simulink subsystem "Subsystem_Driver_BAv01"  (R2022b)
settings: Solver=VariableStepAuto  StartTime=0.0  StopTime=10.0  RelTol=1e-3
undefined symbols (not defined in the file): driver, param, route, weatherSim
libraries: slpidlib x2
settings Model: Creator=giaco  LastModifiedBy=giaco

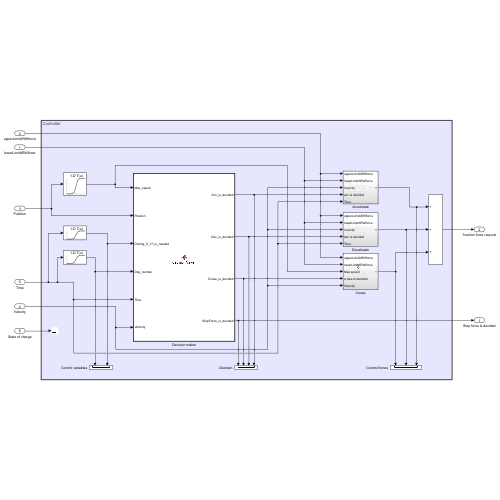
[thumbnail: Simulink's stored preview of the top-level diagram]
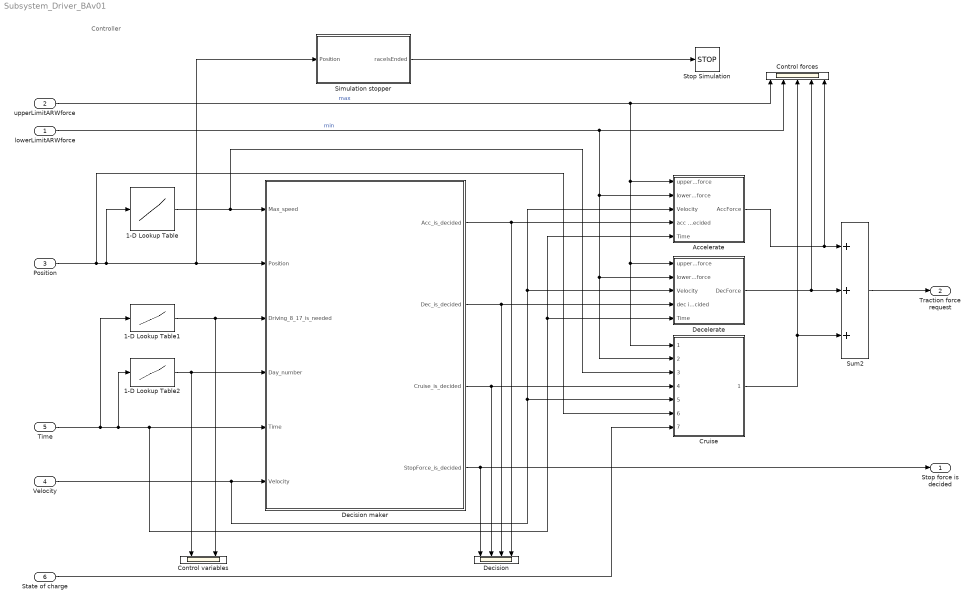
== system Subsystem_Driver_BAv01 ==
  note: Controller
  lowerLimitARWforce : Inport
  upperLimitARWforce : Inport  Port=2
  Position : Inport  Port=3
  Velocity : Inport  Port=4
  Time : Inport  Port=5
  State of charge : Inport  Port=6
  1-D Lookup Table : Lookup_n-D  NumberOfTableDimensions=1  BreakpointsForDimension1=route.dist  Table=route.maxSpeed  InternalRulePriority=Speed  RndMeth=Simplest
  1-D Lookup Table1 : Lookup_n-D  NumberOfTableDimensions=1  BreakpointsForDimension1=weatherSim.irradiance.timeSec  Table=weatherSim.irradiance.driving_8_17_Sec  InternalRulePriority=Speed
  1-D Lookup Table2 : Lookup_n-D  NumberOfTableDimensions=1  BreakpointsForDimension1=weatherSim.irradiance.timeSec  Table=weatherSim.irradiance.dayNumSec  InternalRulePriority=Speed
  Accelerate : Subsystem
  Control forces : Scope  NumInputPorts=5
  Control variables : Scope  NumInputPorts=2
  Cruise : Subsystem  ReferencedSubsystem=Subsystem_Driver_Cruise_BAv01
  Decelerate : Subsystem
  Decision : Scope  NumInputPorts=4
  Decision maker : MATLAB Function  TreatAsAtomicUnit=on
  Simulation stopper : MATLAB Function  TreatAsAtomicUnit=on
  Stop Simulation : Stop
  Sum2 : Sum  Inputs=+++
  Stop force is decided : Outport
  Traction force request : Outport  Port=2
  wires:
  Decision maker/4(StopForce_is_decided) -> Decision/1, Stop force is decided/1
  Accelerate/1(AccForce) -> Control forces/5, Sum2/1
  upperLimitARWforce/1 -> Decelerate/1(upperLimitARWforce), Cruise/1, Accelerate/1(upperLimitARWforce), Control forces/1  "max"
  Sum2/1 -> Traction force request/1
  Velocity/1 -> Decision maker/6(Velocity), Cruise/5, Accelerate/3(Velocity), Decelerate/3(Velocity)
  Decision maker/2(Dec_is_decided) -> Decision/3, Decelerate/4(dec is decided)
  Decision maker/1(Acc_is_decided) -> Decision/4, Accelerate/4(acc is decided)
  lowerLimitARWforce/1 -> Accelerate/2(lowerLimitARWforce), Decelerate/2(lowerLimitARWforce), Cruise/2, Control forces/2  "min"
  1-D Lookup Table/1 -> Decision maker/1(Max_speed), Cruise/3
  Decelerate/1(DecForce) -> Control forces/4, Sum2/2
  Time/1 -> Decision maker/5(Time), Accelerate/5(Time), Decelerate/5(Time), 1-D Lookup Table2/1, 1-D Lookup Table1/1
  Decision maker/3(Cruise_is_decided) -> Cruise/4, Decision/2
  Cruise/1 -> Control forces/3, Sum2/3
  Position/1 -> Decision maker/2(Position), Simulation stopper/1(Position), 1-D Lookup Table/1, Cruise/6
  1-D Lookup Table1/1 -> Control variables/2, Decision maker/3(Driving_8_17_is_needed)
  1-D Lookup Table2/1 -> Decision maker/4(Day_number), Control variables/1
  State of charge/1 -> Cruise/7
  Simulation stopper/1(raceIsEnded) -> Stop Simulation/1

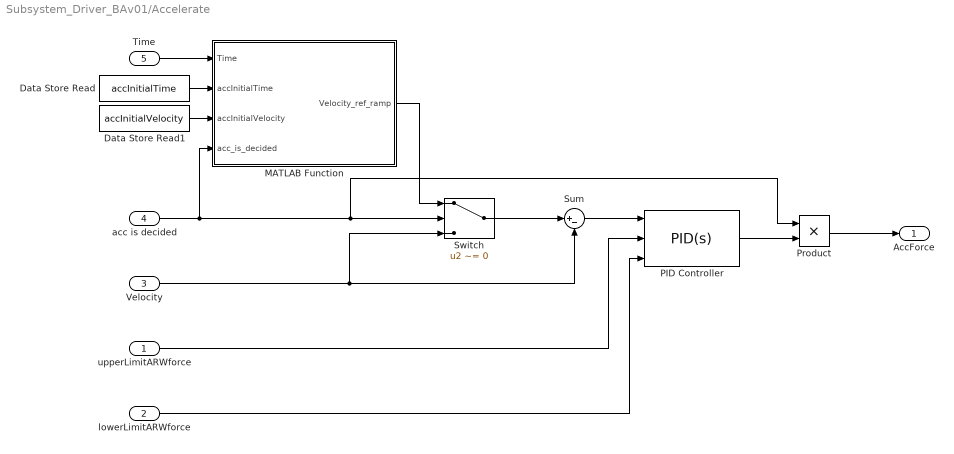
== system Subsystem_Driver_BAv01/Accelerate ==
  upperLimitARWforce : Inport
  lowerLimitARWforce : Inport  Port=2
  Velocity : Inport  Port=3
  acc is decided : Inport  Port=4
  Time : Inport  Port=5
  Data Store Read : DataStoreRead  DataStoreName=accInitialTime  IndexOptions=Index vector (dialog)  Indices=1  OutputSizes=1
  Data Store Read1 : DataStoreRead  DataStoreName=accInitialVelocity  IndexOptions=Index vector (dialog)  Indices=1  OutputSizes=1
  MATLAB Function : MATLAB Function  TreatAsAtomicUnit=on
  PID Controller : slpidlib/PID Controller  Controller=PID  Form=Ideal  TimeDomain=Continuous-time  UseExternalTs=off  SampleTime=-1  IntegratorMethod=Forward Euler  FilterMethod=Forward Euler  ControllerParametersSource=internal  P=4000  I=80/1  UseKiTs=off  D=0  N=100  UseFilter=on  TunerSelectOption=Transfer Function Based (PID Tuner App)  InitialConditionSource=internal  InitialConditionForIntegrator=0  InitialConditionForFilter=0  DifferentiatorICPrevScaledInput=0  ExternalReset=none  TrackingMode=off  Kt=1  LimitOutput=on  SatLimitsSource=external  UpperSaturationLimit=param.motor.maxTorque * param.motor.transmissionRatio / param.suspension.rWheel  LowerSaturationLimit=param.motor.minTorque * param.motor.transmissionRatio / param.suspension.rWheel  LinearizeAsGain=on  AntiWindupMode=clamping  Kb=1  LimitIntegrator=off  UpperIntegratorSaturationLimit=inf  LowerIntegratorSaturationLimit=-inf  POutMin=[]  POutMax=[]  IOutMin=[]  IOutMax=[]  DOutMin=[]  DOutMax=[]  NOutMin=[]  NOutMax=[]  SumOutMin=[]  SumOutMax=[]  SaturationOutMin=[]  SaturationOutMax=[]  PParamMin=[]  PParamMax=[]  IParamMin=[]  IParamMax=[]  DParamMin=[]  DParamMax=[]  NParamMin=[]  NParamMax=[]  KbParamMin=[]  KbParamMax=[]  KtParamMin=[]  KtParamMax=[]  KbOutMin=[]  KbOutMax=[]  KtOutMin=[]  KtOutMax=[]  IntegratorOutMin=[]  IntegratorOutMax=[]  FilterOutMin=[]  FilterOutMax=[]  SumI1OutMin=[]  SumI1OutMax=[]  SumI2OutMin=[]  SumI2OutMax=[]  SumI3OutMin=[]  SumI3OutMax=[]  SumI4OutMin=[]  SumI4OutMax=[]  SumDOutMin=[]  SumDOutMax=[]  DifferentiatorOutMin=[]  DifferentiatorOutMax=[]  FilterDiffOutCoefMin=[]  FilterDiffOutCoefMax=[]  ReciprocalOutMin=[]  ReciprocalOutMax=[]  SumDenOutMin=[]  SumDenOutMax=[]  SumNumOutMin=[]  SumNumOutMax=[]  DivideOutMin=[]  DivideOutMax=[]  UdiffTsProdOutMin=[]  UdiffTsProdOutMax=[]  NTsProdOutMin=[]  NTsProdOutMax=[]  UintegralTsProdOutMin=[]  UintegralTsProdOutMax=[]  UngainTsProdOutMin=[]  UngainTsProdOutMax=[]  ClampingZeroOutDataTypeStr=Inherit: Inherit via back propagation  ClampingZeroOutMin=[]  ClampingZeroOutMax=[]  FilterDenConstantOutDataTypeStr=Inherit: Inherit via back propagation  FilterDenConstantOutMin=[]  FilterDenConstantOutMax=[]  PCopyOutDataTypeStr=Inherit: Inherit via back propagation  PCopyOutMin=[]  PCopyOutMax=[]  NCopyOutDataTypeStr=Inherit: Inherit via back propagation  NCopyOutMin=[]  NCopyOutMax=[]  IntegratorContinuousStateAttributes=''  IntegratorStateMustResolveToSignalObject=off  IntegratorRTWStateStorageClass=Auto  FilterContinuousStateAttributes=''  FilterStateMustResolveToSignalObject=off  FilterRTWStateStorageClass=Auto  ParallelPVariant=Passthrough  IdealPVariant=InternalParameters  IVariant=InternalParameters  DVariant=InternalParameters  IntegratorVariant=Continuous  SatVariant=External  AWVariant=ContClampingIdeal  PCopyVariant=InternalParamsIdeal  TRVariant=Disabled  FdbkBlocksVariant=Forward  IdealPFdbkVariant=Disabled  SatFdbkVariant=Disabled  DerivativeFilterVariant=ContFilter  NVariant=InternalParameters  NCopyVariant=Disabled  FilterICVariant=InternalICsFilter  IntegratorICVariant=InternalICs  ExternalResetVariant=Disabled  TRSumVariant=Passthrough  SumFdbkVariant=Disabled  SumVariant=Sum_PID  TsampFilterVariant=InternalTs  TsampNgainVariant=Passthrough  TsampIntegralVariant=Passthrough  ExternalSaturationOutDataTypeStr=Inherit: Same as second input
  Product : Product
  Sum : Sum  Inputs=|+-
  Switch : Switch  Criteria=u2 ~= 0  SaturateOnIntegerOverflow=off  InputSameDT=off
  AccForce : Outport
  wires:
  acc is decided/1 -> MATLAB Function/4(acc_is_decided), Product/1, Switch/2
  Switch/1 -> Sum/1
  Velocity/1 -> Sum/2, Switch/3
  Sum/1 -> PID Controller/1
  PID Controller/1 -> Product/2
  Product/1 -> AccForce/1
  Time/1 -> MATLAB Function/1(Time)
  MATLAB Function/1(Velocity_ref_ramp) -> Switch/1
  Data Store Read/1 -> MATLAB Function/2(accInitialTime)
  Data Store Read1/1 -> MATLAB Function/3(accInitialVelocity)
  upperLimitARWforce/1 -> PID Controller/2
  lowerLimitARWforce/1 -> PID Controller/3

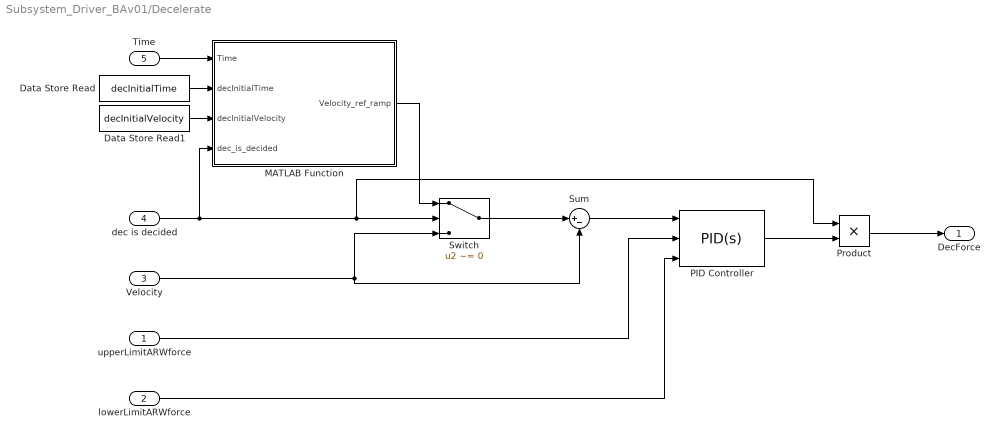
== system Subsystem_Driver_BAv01/Decelerate ==
  upperLimitARWforce : Inport
  lowerLimitARWforce : Inport  Port=2
  Velocity : Inport  Port=3
  dec is decided : Inport  Port=4
  Time : Inport  Port=5
  Data Store Read : DataStoreRead  DataStoreName=decInitialTime  IndexOptions=Index vector (dialog)  Indices=1  OutputSizes=1
  Data Store Read1 : DataStoreRead  DataStoreName=decInitialVelocity  IndexOptions=Index vector (dialog)  Indices=1  OutputSizes=1
  MATLAB Function : MATLAB Function  TreatAsAtomicUnit=on
  PID Controller : slpidlib/PID Controller  Controller=PID  Form=Ideal  TimeDomain=Continuous-time  UseExternalTs=off  SampleTime=-1  IntegratorMethod=Forward Euler  FilterMethod=Forward Euler  ControllerParametersSource=internal  P=4000  I=1/1  UseKiTs=off  D=0  N=100  UseFilter=on  TunerSelectOption=Transfer Function Based (PID Tuner App)  InitialConditionSource=internal  InitialConditionForIntegrator=0  InitialConditionForFilter=0  DifferentiatorICPrevScaledInput=0  ExternalReset=none  TrackingMode=off  Kt=1  LimitOutput=on  SatLimitsSource=external  UpperSaturationLimit=param.motor.maxTorque * param.motor.transmissionRatio / param.suspension.rWheel  LowerSaturationLimit=param.motor.minTorque * param.motor.transmissionRatio / param.suspension.rWheel  LinearizeAsGain=on  AntiWindupMode=clamping  Kb=1  LimitIntegrator=off  UpperIntegratorSaturationLimit=inf  LowerIntegratorSaturationLimit=-inf  POutMin=[]  POutMax=[]  IOutMin=[]  IOutMax=[]  DOutMin=[]  DOutMax=[]  NOutMin=[]  NOutMax=[]  SumOutMin=[]  SumOutMax=[]  SaturationOutMin=[]  SaturationOutMax=[]  PParamMin=[]  PParamMax=[]  IParamMin=[]  IParamMax=[]  DParamMin=[]  DParamMax=[]  NParamMin=[]  NParamMax=[]  KbParamMin=[]  KbParamMax=[]  KtParamMin=[]  KtParamMax=[]  KbOutMin=[]  KbOutMax=[]  KtOutMin=[]  KtOutMax=[]  IntegratorOutMin=[]  IntegratorOutMax=[]  FilterOutMin=[]  FilterOutMax=[]  SumI1OutMin=[]  SumI1OutMax=[]  SumI2OutMin=[]  SumI2OutMax=[]  SumI3OutMin=[]  SumI3OutMax=[]  SumI4OutMin=[]  SumI4OutMax=[]  SumDOutMin=[]  SumDOutMax=[]  DifferentiatorOutMin=[]  DifferentiatorOutMax=[]  FilterDiffOutCoefMin=[]  FilterDiffOutCoefMax=[]  ReciprocalOutMin=[]  ReciprocalOutMax=[]  SumDenOutMin=[]  SumDenOutMax=[]  SumNumOutMin=[]  SumNumOutMax=[]  DivideOutMin=[]  DivideOutMax=[]  UdiffTsProdOutMin=[]  UdiffTsProdOutMax=[]  NTsProdOutMin=[]  NTsProdOutMax=[]  UintegralTsProdOutMin=[]  UintegralTsProdOutMax=[]  UngainTsProdOutMin=[]  UngainTsProdOutMax=[]  ClampingZeroOutDataTypeStr=Inherit: Inherit via back propagation  ClampingZeroOutMin=[]  ClampingZeroOutMax=[]  FilterDenConstantOutDataTypeStr=Inherit: Inherit via back propagation  FilterDenConstantOutMin=[]  FilterDenConstantOutMax=[]  PCopyOutDataTypeStr=Inherit: Inherit via back propagation  PCopyOutMin=[]  PCopyOutMax=[]  NCopyOutDataTypeStr=Inherit: Inherit via back propagation  NCopyOutMin=[]  NCopyOutMax=[]  IntegratorContinuousStateAttributes=''  IntegratorStateMustResolveToSignalObject=off  IntegratorRTWStateStorageClass=Auto  FilterContinuousStateAttributes=''  FilterStateMustResolveToSignalObject=off  FilterRTWStateStorageClass=Auto  ParallelPVariant=Passthrough  IdealPVariant=InternalParameters  IVariant=InternalParameters  DVariant=InternalParameters  IntegratorVariant=Continuous  SatVariant=External  AWVariant=ContClampingIdeal  PCopyVariant=InternalParamsIdeal  TRVariant=Disabled  FdbkBlocksVariant=Forward  IdealPFdbkVariant=Disabled  SatFdbkVariant=Disabled  DerivativeFilterVariant=ContFilter  NVariant=InternalParameters  NCopyVariant=Disabled  FilterICVariant=InternalICsFilter  IntegratorICVariant=InternalICs  ExternalResetVariant=Disabled  TRSumVariant=Passthrough  SumFdbkVariant=Disabled  SumVariant=Sum_PID  TsampFilterVariant=InternalTs  TsampNgainVariant=Passthrough  TsampIntegralVariant=Passthrough  ExternalSaturationOutDataTypeStr=Inherit: Same as second input
  Product : Product
  Sum : Sum  Inputs=|+-
  Switch : Switch  Criteria=u2 ~= 0  SaturateOnIntegerOverflow=off  InputSameDT=off
  DecForce : Outport
  wires:
  dec is decided/1 -> MATLAB Function/4(dec_is_decided), Product/1, Switch/2
  Switch/1 -> Sum/1
  Velocity/1 -> Sum/2, Switch/3
  PID Controller/1 -> Product/2
  Sum/1 -> PID Controller/1
  Product/1 -> DecForce/1
  Time/1 -> MATLAB Function/1(Time)
  Data Store Read1/1 -> MATLAB Function/3(decInitialVelocity)
  MATLAB Function/1(Velocity_ref_ramp) -> Switch/1
  Data Store Read/1 -> MATLAB Function/2(decInitialTime)
  upperLimitARWforce/1 -> PID Controller/2
  lowerLimitARWforce/1 -> PID Controller/3

== matlab function Subsystem_Driver_BAv01/Accelerate/MATLAB Function ==
  data: Time input; Velocity_ref_ramp output; accInitialTime input; accInitialVelocity input; driver parameter; acc_is_decided input
function Velocity_ref_ramp = fcn(Time, accInitialTime, accInitialVelocity, driver, acc_is_decided)

Velocity_ref_ramp = 0;

if acc_is_decided
    Velocity_ref_ramp = driver.accRef .* (Time - accInitialTime) + accInitialVelocity;
end

== matlab function Subsystem_Driver_BAv01/Decelerate/MATLAB Function ==
  data: Time input; Velocity_ref_ramp output; decInitialTime input; decInitialVelocity input; driver parameter; dec_is_decided input
function Velocity_ref_ramp = fcn(Time, decInitialTime, decInitialVelocity, driver, dec_is_decided)

Velocity_ref_ramp = 0;

if dec_is_decided
    Velocity_ref_ramp = driver.decRef .* (Time - decInitialTime) + decInitialVelocity;
end

== matlab function Subsystem_Driver_BAv01/Decision maker ==
  settings: updateMethod=DISCRETE
  data: Max_speed input; Position input; Driving_8_17_is_needed input; Day_number input; Time input; Velocity input; spaceStopIsOver data_store_memory; timeStopIsNeeded data_store_memory; spaceStopIsNeeded data_store_memory; driver parameter; spaceStopNumber data_store_memory; spaceStopIsStarted data_store_memory; Acc_is_decided output; Dec_is_decided output; Cruise_is_decided output; StopForce_is_decided output; spaceStopInitialTime data_store_memory; accInitialTime data_store_memory; accInitialVelocity data_store_memory; decInitialTime data_store_memory; decInitialVelocity data_store_memory; racingDayIsStarted data_store_memory; dayNumber data_store_memory; weatherSim parameter
function [Acc_is_decided, Dec_is_decided, Cruise_is_decided, StopForce_is_decided] = decisionMaker(Max_speed, Position, Driving_8_17_is_needed, Day_number, Time, Velocity, driver, weatherSim)

global racingDayIsStarted
global timeStopIsNeeded
global dayNumber

global spaceStopIsNeeded
global spaceStopIsStarted
global spaceStopIsOver
global spaceStopInitialTime
global spaceStopNumber

global accInitialTime
global accInitialVelocity
global decInitialTime
global decInitialVelocity

Acc_is_decided = false;
Dec_is_decided = false;
Cruise_is_decided = false;
StopForce_is_decided = false;

controlVelocity = min(driver.velRef, Max_speed);

%% Check for stops
% Time stops
stopTime = Time - Velocity ./ driver.decRef;

if ~timeStopIsNeeded && stopTime >= (weatherSim.irradiance.stopTimeSec(Day_number) - 60) %to be sure to stop on time
    timeStopIsNeeded = true;
    decInitialTime = Time; %initialization of time and velocity for ramp controller
    decInitialVelocity = Velocity;
end % if

% Space stops
stopDistance = Position - Velocity.^2 / (2 * driver.decRef);

if ~spaceStopIsNeeded && stopDistance >= driver.stopLocDist(spaceStopNumber)
    spaceStopIsNeeded = true;
    decInitialTime = Time; %initialization of time and velocity for ramp controller
    decInitialVelocity = Velocity;
    
    if spaceStopNumber < length(driver.stopLocDist) %omit last stop: stop simulation
        spaceStopNumber = spaceStopNumber + 1;
    end % if
end % if

%% Check for new racing day
if Driving_8_17_is_needed && Day_number == dayNumber
    racingDayIsStarted = true;
    timeStopIsNeeded = false;
    dayNumber = dayNumber + 1;
end % if

%% Select control options
%% Deceleration
if timeStopIsNeeded
    if Velocity > driver.velRefStop
        Dec_is_decided = true;
    else %if Velocity <= driver.velRefStop
        StopForce_is_decided = true;
        Dec_is_decided = false;
    end % if

elseif spaceStopIsNeeded
    if spaceStopIsStarted
        spaceStopDuration = Time - spaceStopInitialTime;
        if spaceStopDuration >= 30*60
            spaceStopIsNeeded = false;
            spaceStopIsStarted = false;
            spaceStopIsOver = true;
            Acc_is_decided = true;
            accInitialTime = Time;
            accInitialVelocity = Velocity;
        else
            StopForce_is_decided = true;
        end % if
    else
        if Velocity > driver.velRefStop
            Dec_is_decided = true;
        else %if Velocity <= driver.velRefStop
            spaceStopIsStarted = true;
            spaceStopInitialTime = Time;
            StopForce_is_decided = true;
        end % if
    end % if

%% Acceleration
elseif racingDayIsStarted
    if Velocity < 0.9 * controlVelocity
        Acc_is_decided = true;
    else %if Velocity >= 0.9 * controlVelocity
        Cruise_is_decided = true;
        racingDayIsStarted = false;
    end % if

elseif spaceStopIsOver
    if Velocity < 0.9 * controlVelocity
        Acc_is_decided = true;
    else %if Velocity >= 0.9 * controlVelocity
        Cruise_is_decided = true;
        spaceStopIsOver = false;
    end % if

else
    Cruise_is_decided = true;
end % if

== matlab function Subsystem_Driver_BAv01/Simulation stopper ==
  data: Position input; raceIsEnded output; driver parameter
function raceIsEnded = simulationStopper(Position, driver)

raceIsEnded = false;

if Position >= driver.stopLocDist(end)
    raceIsEnded = true;
end % if
